simulink model "overalldesign_change_down"  (R2025b)
settings: Solver=ode4  StartTime=0.0  StopTime=1200  FixedStep=0.01  MaxStep=0.01  RelTol=1e-4
PreLoadFcn:
  | % Component data matrix: [present, weight_kg, MX_kgmm, MY_kgmm, MZ_kgmm]
  | % Rows 1-28 correspond to Excel rows 2-29
  | comp_data_mat = [
  |   1, 80,     147543.64,  -0.88,    -1622.36;    % 底盘
  |   1, 60,      73274.04, -169.26,    3359.46;    % 轮胎
  |   0,  0,             0,       0,         0;    % 前后桥(不在位)
  |   1, 45,      99639.05,  -0.495,   35241.39;    % 蒙皮
  |   1, 159,    308512.15, -0.0298,   72044.97;    % 结构骨架
  |   1, 93,     214584.20,  -1.023,   85225.94;    % 折叠机构
  |   1, 113.92, 269830.46, -1.2531,  107552.44;    % 支臂
  |   1, 45,       1371.65, -531.27,   17662.14;    % 内饰
  |   1, 13.86,   34638.76, -0.1525,   13254.18;    % 电机底座
  |   1, 30,      69816.09,   -0.33,   26989.32;    % 飞行体
  |   1, 316,    803427.47,       0,   33092.78;    % 动力电池1
  |   0, 316,            0,       0,         0;    % 动力电池2(不在位)
  |   1, 30,      75059.94,    0.21,   37410.81;    % 旋翼
  |   1, 141,    353019.16,  -1.551,  161459.10;    % 电机
  |   1, 33,      82253.26,   -0.33,   27077.13;    % 电调
  |   1, 15,             0,       0,         0;    % PDU
  |   0, 10,             0,       0,         0;    % 导线(不在位)
  |   0,  0,             0,       0,         0;    % (空)
  |   0, 90,             0,       0,         0;    % 左商载(不在位)
  |   0, 90,             0,       0,         0;    % 右商载(不在位)
  |   0, 32,             0,       0,         0;    % 飞控运控(不在位)
  | 
  | ];
  | % Lift center [X; Y; Z] in mm
  | lift_center_vec = [2506.477; 0; 1258.273];
  | % Route parameters are set directly in top-level Constant blocks:
  | %   route_mode, takeoff, hover, line_cruise, circle_cruise, land
model workspace (MAT data in the model file):
  CS_duct_lift_slew_rate = 7031250
  CS_main_rotor_slew_rate = 1567.1641791
  CS_max_acc_xy = 5
  CS_max_acc_z_down = 5
  CS_max_acc_z_up = 5
  CS_max_jerk_xy = 20
  CS_max_jerk_z_down = 20
  CS_max_jerk_z_up = 20
  CS_max_vel_xy = 20
  CS_max_vel_z_down = 20
  CS_max_vel_z_up = 20
  CS_motor_tau_duct = 0.07
  CS_motor_tau_main = 0.336
  Kd_rate_rp = 12
  Kd_rate_y = 8
  Kd_vel_xy = 1.5
  Kd_vel_z = 1
  Ki_rate_rp = 4
  Ki_rate_y = 10
  Ki_vel_xy = 0.02
  Ki_vel_z = 0.05
  Kp_att_rp = 2.5
  Kp_att_tilt = 2.5
  Kp_att_y = 1.5
  Kp_att_yaw = 1.5
  Kp_pos_xy = 0.4
  Kp_pos_z = 1
  Kp_rate_rp = 300
  Kp_rate_y = 200
  Kp_vel_xy = 1.5
  Kp_vel_z = 1.5
  P : object (value not decoded)
  T_hover = 11772
  V_descent = []
  W_hover = 1194
  W_margin = 1600
  cg_offset_m = [0.038293; -0.0063; 0.28227]
  cg_x_delta_m = 0
  climbRate_mps = 5
  cruiseSpeed_mps = 20
  descentRate_mps = 5
  duct_dir = [0  -1  0; 0  1  0]
  duct_pos_0 = [3  0  0; 3  0  0]
  fault_id = 0
  fault_mask = [0; 0; 0; 0; 0; 0; 0; 0]
  hover_x = 0
  hover_y = 0
  hover_yaw = 0
  hover_z = -120
  inertia_kgm2 = [3959.6  0  0; 0  3041.4  0; 0  0  2640.2]
  kF = 0.0013767
  kF_duct = 4.54e-05
  kM = 0.000164967
  kM_coeff = 1.72621225e-05
  kM_duct = 4.896e-06
  kM_duct_coeff = 5.12708e-07
  k_yaw_weight = 0.5
  mass_kg = 1200
  motor_coord = [2.624 2.624 0 0 -2.599 -2.599 3 3 -2.228 2.228 -2.235 2.235 ... (24 elements, 8x3)]
  motor_dir = [1; -1; -1; 1; 1; -1]
  motor_efficiency = 0.9016
  motor_pos_0 = [2.624 2.624 0 0 -2.599 -2.599 -2.228 2.228 -2.235 2.235 -2.231 2.231 ... (18 elements, 6x3)]
  offline_opt_applyBestToModel = 1
  offline_opt_maxEvaluations = 10
  offline_opt_method = 'auto'
  offline_opt_saveBestToModel = 0
  offline_opt_updateDiagramAfterBest = 1
  perf_battery_Wh = 80000
  perf_blade_num = 2
  perf_chord_avg = 0.18
  perf_mass_kg = 1200
  perf_rho = 1.225
  perf_rotor_num = 6
  perf_rotor_radius = 1.3
  perf_usable_ratio = 0.8
  speed_max_radps = 1750
  tau_limit_rp = 2000
  tau_limit_y = 1000
  thrust_degrade = 0.7
libraries: slpidlib x6, aerolibprivatev1p5 x1, dspnetwork x1
(part 2 of 2)

== system overalldesign_change_down/Flight_Simulation/controller/Rate_Controller ==
  p_sp : Inport
  q_sp : Inport  Port=2
  r_sp : Inport  Port=3
  cur_p : Inport  Port=4
  cur_q : Inport  Port=5
  cur_r : Inport  Port=6
  PID_RatePitch : slpidlib/PID Controller  Controller=PID  Form=Parallel  TimeDomain=Continuous-time  UseExternalTs=off  SampleTime=-1  IntegratorMethod=Forward Euler  FilterMethod=Forward Euler  ControllerParametersSource=internal  P=Kp_rate_rp  I=Ki_rate_rp  UseKiTs=off  D=Kd_rate_rp  UseExternalDerivativeSource=off  N=100  UseFilter=on  TunerSelectOption=Transfer Function Based (PID Tuner App)  InitialConditionSource=internal  InitialConditionForIntegrator=0  InitialConditionForFilter=0  DifferentiatorICPrevScaledInput=0  ExternalReset=none  TrackingMode=off  Kt=1  LimitOutput=on  SatLimitsSource=internal  UpperSaturationLimit=tau_limit_rp  LowerSaturationLimit=-tau_limit_rp  LinearizeAsGain=on  AntiWindupMode=clamping  Kb=1  LimitIntegrator=on  UpperIntegratorSaturationLimit=tau_limit_rp  LowerIntegratorSaturationLimit=-tau_limit_rp  POutMin=[]  POutMax=[]  IOutMin=[]  IOutMax=[]  DOutMin=[]  DOutMax=[]  NOutMin=[]  NOutMax=[]  SumOutMin=[]  SumOutMax=[]  SaturationOutMin=[]  SaturationOutMax=[]  PParamMin=[]  PParamMax=[]  IParamMin=[]  IParamMax=[]  DParamMin=[]  DParamMax=[]  NParamMin=[]  NParamMax=[]  KbParamMin=[]  KbParamMax=[]  KtParamMin=[]  KtParamMax=[]  KbOutMin=[]  KbOutMax=[]  KtOutMin=[]  KtOutMax=[]  IntegratorOutMin=[]  IntegratorOutMax=[]  FilterOutMin=[]  FilterOutMax=[]  SumI1OutMin=[]  SumI1OutMax=[]  SumI2OutMin=[]  SumI2OutMax=[]  SumI3OutMin=[]  SumI3OutMax=[]  SumI4OutMin=[]  SumI4OutMax=[]  SumDOutMin=[]  SumDOutMax=[]  DifferentiatorOutMin=[]  DifferentiatorOutMax=[]  FilterDiffOutCoefMin=[]  FilterDiffOutCoefMax=[]  ReciprocalOutMin=[]  ReciprocalOutMax=[]  SumDenOutMin=[]  SumDenOutMax=[]  SumNumOutMin=[]  SumNumOutMax=[]  DivideOutMin=[]  DivideOutMax=[]  UdiffTsProdOutMin=[]  UdiffTsProdOutMax=[]  NTsProdOutMin=[]  NTsProdOutMax=[]  UintegralTsProdOutMin=[]  UintegralTsProdOutMax=[]  UngainTsProdOutMin=[]  UngainTsProdOutMax=[]  ClampingZeroOutDataTypeStr=Inherit: Inherit via back propagation  ClampingZeroOutMin=[]  ClampingZeroOutMax=[]  FilterDenConstantOutDataTypeStr=Inherit: Inherit via back propagation  FilterDenConstantOutMin=[]  FilterDenConstantOutMax=[]  PCopyOutDataTypeStr=Inherit: Inherit via back propagation  PCopyOutMin=[]  PCopyOutMax=[]  NCopyOutDataTypeStr=Inherit: Inherit via back propagation  NCopyOutMin=[]  NCopyOutMax=[]  IntegratorContinuousStateAttributes=''  IntegratorStateMustResolveToSignalObject=off  IntegratorRTWStateStorageClass=Auto  FilterContinuousStateAttributes=''  FilterStateMustResolveToSignalObject=off  FilterRTWStateStorageClass=Auto  ParallelPVariant=InternalParameters  IdealPVariant=Disabled  IVariant=InternalParameters  DVariant=InternalParameters  IntegratorVariant=Continuous  SatVariant=Enabled  AWVariant=ContClampingParallel  PCopyVariant=Disabled  TRVariant=Disabled  FdbkBlocksVariant=Forward  IdealPFdbkVariant=Disabled  SatFdbkVariant=Disabled  DerivativeFilterVariant=ContFilter  NVariant=InternalParameters  NCopyVariant=Disabled  FilterICVariant=InternalICsFilter  IntegratorICVariant=InternalICs  ExternalResetVariant=Disabled  TRSumVariant=Passthrough  SumFdbkVariant=Disabled  SumVariant=Sum_PID  TsampFilterVariant=InternalTs  TsampNgainVariant=Passthrough  TsampIntegralVariant=Disabled_SignalSpec  ExternalSaturationOutDataTypeStr=Inherit: Same as second input  DerivativeSourceVariant=ErrorSignal  PreIntVariant=InternalPreInt
  PID_RateRoll : slpidlib/PID Controller  Controller=PID  Form=Parallel  TimeDomain=Continuous-time  UseExternalTs=off  SampleTime=-1  IntegratorMethod=Forward Euler  FilterMethod=Forward Euler  ControllerParametersSource=internal  P=Kp_rate_rp  I=Ki_rate_rp  UseKiTs=off  D=Kd_rate_rp  UseExternalDerivativeSource=off  N=100  UseFilter=on  TunerSelectOption=Transfer Function Based (PID Tuner App)  InitialConditionSource=internal  InitialConditionForIntegrator=0  InitialConditionForFilter=0  DifferentiatorICPrevScaledInput=0  ExternalReset=none  TrackingMode=off  Kt=1  LimitOutput=on  SatLimitsSource=internal  UpperSaturationLimit=tau_limit_rp  LowerSaturationLimit=-tau_limit_rp  LinearizeAsGain=on  AntiWindupMode=clamping  Kb=1  LimitIntegrator=on  UpperIntegratorSaturationLimit=tau_limit_rp  LowerIntegratorSaturationLimit=-tau_limit_rp  POutMin=[]  POutMax=[]  IOutMin=[]  IOutMax=[]  DOutMin=[]  DOutMax=[]  NOutMin=[]  NOutMax=[]  SumOutMin=[]  SumOutMax=[]  SaturationOutMin=[]  SaturationOutMax=[]  PParamMin=[]  PParamMax=[]  IParamMin=[]  IParamMax=[]  DParamMin=[]  DParamMax=[]  NParamMin=[]  NParamMax=[]  KbParamMin=[]  KbParamMax=[]  KtParamMin=[]  KtParamMax=[]  KbOutMin=[]  KbOutMax=[]  KtOutMin=[]  KtOutMax=[]  IntegratorOutMin=[]  IntegratorOutMax=[]  FilterOutMin=[]  FilterOutMax=[]  SumI1OutMin=[]  SumI1OutMax=[]  SumI2OutMin=[]  SumI2OutMax=[]  SumI3OutMin=[]  SumI3OutMax=[]  SumI4OutMin=[]  SumI4OutMax=[]  SumDOutMin=[]  SumDOutMax=[]  DifferentiatorOutMin=[]  DifferentiatorOutMax=[]  FilterDiffOutCoefMin=[]  FilterDiffOutCoefMax=[]  ReciprocalOutMin=[]  ReciprocalOutMax=[]  SumDenOutMin=[]  SumDenOutMax=[]  SumNumOutMin=[]  SumNumOutMax=[]  DivideOutMin=[]  DivideOutMax=[]  UdiffTsProdOutMin=[]  UdiffTsProdOutMax=[]  NTsProdOutMin=[]  NTsProdOutMax=[]  UintegralTsProdOutMin=[]  UintegralTsProdOutMax=[]  UngainTsProdOutMin=[]  UngainTsProdOutMax=[]  ClampingZeroOutDataTypeStr=Inherit: Inherit via back propagation  ClampingZeroOutMin=[]  ClampingZeroOutMax=[]  FilterDenConstantOutDataTypeStr=Inherit: Inherit via back propagation  FilterDenConstantOutMin=[]  FilterDenConstantOutMax=[]  PCopyOutDataTypeStr=Inherit: Inherit via back propagation  PCopyOutMin=[]  PCopyOutMax=[]  NCopyOutDataTypeStr=Inherit: Inherit via back propagation  NCopyOutMin=[]  NCopyOutMax=[]  IntegratorContinuousStateAttributes=''  IntegratorStateMustResolveToSignalObject=off  IntegratorRTWStateStorageClass=Auto  FilterContinuousStateAttributes=''  FilterStateMustResolveToSignalObject=off  FilterRTWStateStorageClass=Auto  ParallelPVariant=InternalParameters  IdealPVariant=Disabled  IVariant=InternalParameters  DVariant=InternalParameters  IntegratorVariant=Continuous  SatVariant=Enabled  AWVariant=ContClampingParallel  PCopyVariant=Disabled  TRVariant=Disabled  FdbkBlocksVariant=Forward  IdealPFdbkVariant=Disabled  SatFdbkVariant=Disabled  DerivativeFilterVariant=ContFilter  NVariant=InternalParameters  NCopyVariant=Disabled  FilterICVariant=InternalICsFilter  IntegratorICVariant=InternalICs  ExternalResetVariant=Disabled  TRSumVariant=Passthrough  SumFdbkVariant=Disabled  SumVariant=Sum_PID  TsampFilterVariant=InternalTs  TsampNgainVariant=Passthrough  TsampIntegralVariant=Disabled_SignalSpec  ExternalSaturationOutDataTypeStr=Inherit: Same as second input  DerivativeSourceVariant=ErrorSignal  PreIntVariant=InternalPreInt
  PID_RateYaw : slpidlib/PID Controller  Controller=PID  Form=Parallel  TimeDomain=Continuous-time  UseExternalTs=off  SampleTime=-1  IntegratorMethod=Forward Euler  FilterMethod=Forward Euler  ControllerParametersSource=internal  P=Kp_rate_y  I=Ki_rate_y  UseKiTs=off  D=Kd_rate_y  UseExternalDerivativeSource=off  N=100  UseFilter=on  TunerSelectOption=Transfer Function Based (PID Tuner App)  InitialConditionSource=internal  InitialConditionForIntegrator=0  InitialConditionForFilter=0  DifferentiatorICPrevScaledInput=0  ExternalReset=none  TrackingMode=off  Kt=1  LimitOutput=on  SatLimitsSource=internal  UpperSaturationLimit=tau_limit_y  LowerSaturationLimit=-tau_limit_y  LinearizeAsGain=on  AntiWindupMode=clamping  Kb=1  LimitIntegrator=on  UpperIntegratorSaturationLimit=tau_limit_y  LowerIntegratorSaturationLimit=-tau_limit_y  POutMin=[]  POutMax=[]  IOutMin=[]  IOutMax=[]  DOutMin=[]  DOutMax=[]  NOutMin=[]  NOutMax=[]  SumOutMin=[]  SumOutMax=[]  SaturationOutMin=[]  SaturationOutMax=[]  PParamMin=[]  PParamMax=[]  IParamMin=[]  IParamMax=[]  DParamMin=[]  DParamMax=[]  NParamMin=[]  NParamMax=[]  KbParamMin=[]  KbParamMax=[]  KtParamMin=[]  KtParamMax=[]  KbOutMin=[]  KbOutMax=[]  KtOutMin=[]  KtOutMax=[]  IntegratorOutMin=[]  IntegratorOutMax=[]  FilterOutMin=[]  FilterOutMax=[]  SumI1OutMin=[]  SumI1OutMax=[]  SumI2OutMin=[]  SumI2OutMax=[]  SumI3OutMin=[]  SumI3OutMax=[]  SumI4OutMin=[]  SumI4OutMax=[]  SumDOutMin=[]  SumDOutMax=[]  DifferentiatorOutMin=[]  DifferentiatorOutMax=[]  FilterDiffOutCoefMin=[]  FilterDiffOutCoefMax=[]  ReciprocalOutMin=[]  ReciprocalOutMax=[]  SumDenOutMin=[]  SumDenOutMax=[]  SumNumOutMin=[]  SumNumOutMax=[]  DivideOutMin=[]  DivideOutMax=[]  UdiffTsProdOutMin=[]  UdiffTsProdOutMax=[]  NTsProdOutMin=[]  NTsProdOutMax=[]  UintegralTsProdOutMin=[]  UintegralTsProdOutMax=[]  UngainTsProdOutMin=[]  UngainTsProdOutMax=[]  ClampingZeroOutDataTypeStr=Inherit: Inherit via back propagation  ClampingZeroOutMin=[]  ClampingZeroOutMax=[]  FilterDenConstantOutDataTypeStr=Inherit: Inherit via back propagation  FilterDenConstantOutMin=[]  FilterDenConstantOutMax=[]  PCopyOutDataTypeStr=Inherit: Inherit via back propagation  PCopyOutMin=[]  PCopyOutMax=[]  NCopyOutDataTypeStr=Inherit: Inherit via back propagation  NCopyOutMin=[]  NCopyOutMax=[]  IntegratorContinuousStateAttributes=''  IntegratorStateMustResolveToSignalObject=off  IntegratorRTWStateStorageClass=Auto  FilterContinuousStateAttributes=''  FilterStateMustResolveToSignalObject=off  FilterRTWStateStorageClass=Auto  ParallelPVariant=InternalParameters  IdealPVariant=Disabled  IVariant=InternalParameters  DVariant=InternalParameters  IntegratorVariant=Continuous  SatVariant=Enabled  AWVariant=ContClampingParallel  PCopyVariant=Disabled  TRVariant=Disabled  FdbkBlocksVariant=Forward  IdealPFdbkVariant=Disabled  SatFdbkVariant=Disabled  DerivativeFilterVariant=ContFilter  NVariant=InternalParameters  NCopyVariant=Disabled  FilterICVariant=InternalICsFilter  IntegratorICVariant=InternalICs  ExternalResetVariant=Disabled  TRSumVariant=Passthrough  SumFdbkVariant=Disabled  SumVariant=Sum_PID  TsampFilterVariant=InternalTs  TsampNgainVariant=Passthrough  TsampIntegralVariant=Disabled_SignalSpec  ExternalSaturationOutDataTypeStr=Inherit: Same as second input  DerivativeSourceVariant=ErrorSignal  PreIntVariant=InternalPreInt
  Sum_Pitch : Sum  Inputs=+-
  Sum_Roll : Sum  Inputs=+-
  Sum_Yaw : Sum  Inputs=+-
  tau_x : Outport
  tau_y : Outport  Port=2
  tau_z : Outport  Port=3
  wires:
  Sum_Yaw/1 -> PID_RateYaw/1
  p_sp/1 -> Sum_Roll/1
  cur_q/1 -> Sum_Pitch/2
  cur_p/1 -> Sum_Roll/2
  PID_RateYaw/1 -> tau_z/1
  r_sp/1 -> Sum_Yaw/1
  cur_r/1 -> Sum_Yaw/2
  q_sp/1 -> Sum_Pitch/1
  Sum_Roll/1 -> PID_RateRoll/1
  Sum_Pitch/1 -> PID_RatePitch/1
  PID_RateRoll/1 -> tau_x/1
  PID_RatePitch/1 -> tau_y/1

== system overalldesign_change_down/Flight_Simulation/controller/Velocity_Controller ==
  vx_sp : Inport
  vy_sp : Inport  Port=2
  vz_sp : Inport  Port=3
  cur_vx : Inport  Port=4
  cur_vy : Inport  Port=5
  cur_vz : Inport  Port=6
  AccelJerkLimit_X : RateLimiter  RisingSlewLimit=CS_max_jerk_xy  FallingSlewLimit=-CS_max_jerk_xy  SampleTimeMode=inherited
  AccelJerkLimit_Y : RateLimiter  RisingSlewLimit=CS_max_jerk_xy  FallingSlewLimit=-CS_max_jerk_xy  SampleTimeMode=inherited
  AccelJerkLimit_Z : RateLimiter  RisingSlewLimit=CS_max_jerk_z_up  FallingSlewLimit=-CS_max_jerk_z_down  SampleTimeMode=inherited
  PID_VelX : slpidlib/PID Controller  Controller=PID  Form=Parallel  TimeDomain=Continuous-time  UseExternalTs=off  SampleTime=-1  IntegratorMethod=Forward Euler  FilterMethod=Forward Euler  ControllerParametersSource=internal  P=Kp_vel_xy  I=Ki_vel_xy  UseKiTs=off  D=Kd_vel_xy  UseExternalDerivativeSource=off  N=10  UseFilter=on  TunerSelectOption=Transfer Function Based (PID Tuner App)  InitialConditionSource=internal  InitialConditionForIntegrator=0  InitialConditionForFilter=0  DifferentiatorICPrevScaledInput=0  ExternalReset=none  TrackingMode=off  Kt=1  LimitOutput=on  SatLimitsSource=internal  UpperSaturationLimit=CS_max_acc_xy  LowerSaturationLimit=-CS_max_acc_xy  LinearizeAsGain=on  AntiWindupMode=clamping  Kb=1  LimitIntegrator=on  UpperIntegratorSaturationLimit=5  LowerIntegratorSaturationLimit=-5  POutMin=[]  POutMax=[]  IOutMin=[]  IOutMax=[]  DOutMin=[]  DOutMax=[]  NOutMin=[]  NOutMax=[]  SumOutMin=[]  SumOutMax=[]  SaturationOutMin=[]  SaturationOutMax=[]  PParamMin=[]  PParamMax=[]  IParamMin=[]  IParamMax=[]  DParamMin=[]  DParamMax=[]  NParamMin=[]  NParamMax=[]  KbParamMin=[]  KbParamMax=[]  KtParamMin=[]  KtParamMax=[]  KbOutMin=[]  KbOutMax=[]  KtOutMin=[]  KtOutMax=[]  IntegratorOutMin=[]  IntegratorOutMax=[]  FilterOutMin=[]  FilterOutMax=[]  SumI1OutMin=[]  SumI1OutMax=[]  SumI2OutMin=[]  SumI2OutMax=[]  SumI3OutMin=[]  SumI3OutMax=[]  SumI4OutMin=[]  SumI4OutMax=[]  SumDOutMin=[]  SumDOutMax=[]  DifferentiatorOutMin=[]  DifferentiatorOutMax=[]  FilterDiffOutCoefMin=[]  FilterDiffOutCoefMax=[]  ReciprocalOutMin=[]  ReciprocalOutMax=[]  SumDenOutMin=[]  SumDenOutMax=[]  SumNumOutMin=[]  SumNumOutMax=[]  DivideOutMin=[]  DivideOutMax=[]  UdiffTsProdOutMin=[]  UdiffTsProdOutMax=[]  NTsProdOutMin=[]  NTsProdOutMax=[]  UintegralTsProdOutMin=[]  UintegralTsProdOutMax=[]  UngainTsProdOutMin=[]  UngainTsProdOutMax=[]  ClampingZeroOutDataTypeStr=Inherit: Inherit via back propagation  ClampingZeroOutMin=[]  ClampingZeroOutMax=[]  FilterDenConstantOutDataTypeStr=Inherit: Inherit via back propagation  FilterDenConstantOutMin=[]  FilterDenConstantOutMax=[]  PCopyOutDataTypeStr=Inherit: Inherit via back propagation  PCopyOutMin=[]  PCopyOutMax=[]  NCopyOutDataTypeStr=Inherit: Inherit via back propagation  NCopyOutMin=[]  NCopyOutMax=[]  IntegratorContinuousStateAttributes=''  IntegratorStateMustResolveToSignalObject=off  IntegratorRTWStateStorageClass=Auto  FilterContinuousStateAttributes=''  FilterStateMustResolveToSignalObject=off  FilterRTWStateStorageClass=Auto  ParallelPVariant=InternalParameters  IdealPVariant=Disabled  IVariant=InternalParameters  DVariant=InternalParameters  IntegratorVariant=Continuous  SatVariant=Enabled  AWVariant=ContClampingParallel  PCopyVariant=Disabled  TRVariant=Disabled  FdbkBlocksVariant=Forward  IdealPFdbkVariant=Disabled  SatFdbkVariant=Disabled  DerivativeFilterVariant=ContFilter  NVariant=InternalParameters  NCopyVariant=Disabled  FilterICVariant=InternalICsFilter  IntegratorICVariant=InternalICs  ExternalResetVariant=Disabled  TRSumVariant=Passthrough  SumFdbkVariant=Disabled  SumVariant=Sum_PID  TsampFilterVariant=InternalTs  TsampNgainVariant=Passthrough  TsampIntegralVariant=Disabled_SignalSpec  ExternalSaturationOutDataTypeStr=Inherit: Same as second input  DerivativeSourceVariant=ErrorSignal  PreIntVariant=InternalPreInt
  PID_VelY : slpidlib/PID Controller  Controller=PID  Form=Parallel  TimeDomain=Continuous-time  UseExternalTs=off  SampleTime=-1  IntegratorMethod=Forward Euler  FilterMethod=Forward Euler  ControllerParametersSource=internal  P=Kp_vel_xy  I=Ki_vel_xy  UseKiTs=off  D=Kd_vel_xy  UseExternalDerivativeSource=off  N=10  UseFilter=on  TunerSelectOption=Transfer Function Based (PID Tuner App)  InitialConditionSource=internal  InitialConditionForIntegrator=0  InitialConditionForFilter=0  DifferentiatorICPrevScaledInput=0  ExternalReset=none  TrackingMode=off  Kt=1  LimitOutput=on  SatLimitsSource=internal  UpperSaturationLimit=CS_max_acc_xy  LowerSaturationLimit=-CS_max_acc_xy  LinearizeAsGain=on  AntiWindupMode=clamping  Kb=1  LimitIntegrator=on  UpperIntegratorSaturationLimit=5  LowerIntegratorSaturationLimit=-5  POutMin=[]  POutMax=[]  IOutMin=[]  IOutMax=[]  DOutMin=[]  DOutMax=[]  NOutMin=[]  NOutMax=[]  SumOutMin=[]  SumOutMax=[]  SaturationOutMin=[]  SaturationOutMax=[]  PParamMin=[]  PParamMax=[]  IParamMin=[]  IParamMax=[]  DParamMin=[]  DParamMax=[]  NParamMin=[]  NParamMax=[]  KbParamMin=[]  KbParamMax=[]  KtParamMin=[]  KtParamMax=[]  KbOutMin=[]  KbOutMax=[]  KtOutMin=[]  KtOutMax=[]  IntegratorOutMin=[]  IntegratorOutMax=[]  FilterOutMin=[]  FilterOutMax=[]  SumI1OutMin=[]  SumI1OutMax=[]  SumI2OutMin=[]  SumI2OutMax=[]  SumI3OutMin=[]  SumI3OutMax=[]  SumI4OutMin=[]  SumI4OutMax=[]  SumDOutMin=[]  SumDOutMax=[]  DifferentiatorOutMin=[]  DifferentiatorOutMax=[]  FilterDiffOutCoefMin=[]  FilterDiffOutCoefMax=[]  ReciprocalOutMin=[]  ReciprocalOutMax=[]  SumDenOutMin=[]  SumDenOutMax=[]  SumNumOutMin=[]  SumNumOutMax=[]  DivideOutMin=[]  DivideOutMax=[]  UdiffTsProdOutMin=[]  UdiffTsProdOutMax=[]  NTsProdOutMin=[]  NTsProdOutMax=[]  UintegralTsProdOutMin=[]  UintegralTsProdOutMax=[]  UngainTsProdOutMin=[]  UngainTsProdOutMax=[]  ClampingZeroOutDataTypeStr=Inherit: Inherit via back propagation  ClampingZeroOutMin=[]  ClampingZeroOutMax=[]  FilterDenConstantOutDataTypeStr=Inherit: Inherit via back propagation  FilterDenConstantOutMin=[]  FilterDenConstantOutMax=[]  PCopyOutDataTypeStr=Inherit: Inherit via back propagation  PCopyOutMin=[]  PCopyOutMax=[]  NCopyOutDataTypeStr=Inherit: Inherit via back propagation  NCopyOutMin=[]  NCopyOutMax=[]  IntegratorContinuousStateAttributes=''  IntegratorStateMustResolveToSignalObject=off  IntegratorRTWStateStorageClass=Auto  FilterContinuousStateAttributes=''  FilterStateMustResolveToSignalObject=off  FilterRTWStateStorageClass=Auto  ParallelPVariant=InternalParameters  IdealPVariant=Disabled  IVariant=InternalParameters  DVariant=InternalParameters  IntegratorVariant=Continuous  SatVariant=Enabled  AWVariant=ContClampingParallel  PCopyVariant=Disabled  TRVariant=Disabled  FdbkBlocksVariant=Forward  IdealPFdbkVariant=Disabled  SatFdbkVariant=Disabled  DerivativeFilterVariant=ContFilter  NVariant=InternalParameters  NCopyVariant=Disabled  FilterICVariant=InternalICsFilter  IntegratorICVariant=InternalICs  ExternalResetVariant=Disabled  TRSumVariant=Passthrough  SumFdbkVariant=Disabled  SumVariant=Sum_PID  TsampFilterVariant=InternalTs  TsampNgainVariant=Passthrough  TsampIntegralVariant=Disabled_SignalSpec  ExternalSaturationOutDataTypeStr=Inherit: Same as second input  DerivativeSourceVariant=ErrorSignal  PreIntVariant=InternalPreInt
  PID_VelZ : slpidlib/PID Controller  Controller=PID  Form=Parallel  TimeDomain=Continuous-time  UseExternalTs=off  SampleTime=-1  IntegratorMethod=Forward Euler  FilterMethod=Forward Euler  ControllerParametersSource=internal  P=Kp_vel_z  I=Ki_vel_z  UseKiTs=off  D=Kd_vel_z  UseExternalDerivativeSource=off  N=10  UseFilter=on  TunerSelectOption=Transfer Function Based (PID Tuner App)  InitialConditionSource=internal  InitialConditionForIntegrator=0  InitialConditionForFilter=0  DifferentiatorICPrevScaledInput=0  ExternalReset=none  TrackingMode=off  Kt=1  LimitOutput=on  SatLimitsSource=internal  UpperSaturationLimit=CS_max_acc_z_up  LowerSaturationLimit=-CS_max_acc_z_down  LinearizeAsGain=on  AntiWindupMode=clamping  Kb=1  LimitIntegrator=on  UpperIntegratorSaturationLimit=5  LowerIntegratorSaturationLimit=-5  POutMin=[]  POutMax=[]  IOutMin=[]  IOutMax=[]  DOutMin=[]  DOutMax=[]  NOutMin=[]  NOutMax=[]  SumOutMin=[]  SumOutMax=[]  SaturationOutMin=[]  SaturationOutMax=[]  PParamMin=[]  PParamMax=[]  IParamMin=[]  IParamMax=[]  DParamMin=[]  DParamMax=[]  NParamMin=[]  NParamMax=[]  KbParamMin=[]  KbParamMax=[]  KtParamMin=[]  KtParamMax=[]  KbOutMin=[]  KbOutMax=[]  KtOutMin=[]  KtOutMax=[]  IntegratorOutMin=[]  IntegratorOutMax=[]  FilterOutMin=[]  FilterOutMax=[]  SumI1OutMin=[]  SumI1OutMax=[]  SumI2OutMin=[]  SumI2OutMax=[]  SumI3OutMin=[]  SumI3OutMax=[]  SumI4OutMin=[]  SumI4OutMax=[]  SumDOutMin=[]  SumDOutMax=[]  DifferentiatorOutMin=[]  DifferentiatorOutMax=[]  FilterDiffOutCoefMin=[]  FilterDiffOutCoefMax=[]  ReciprocalOutMin=[]  ReciprocalOutMax=[]  SumDenOutMin=[]  SumDenOutMax=[]  SumNumOutMin=[]  SumNumOutMax=[]  DivideOutMin=[]  DivideOutMax=[]  UdiffTsProdOutMin=[]  UdiffTsProdOutMax=[]  NTsProdOutMin=[]  NTsProdOutMax=[]  UintegralTsProdOutMin=[]  UintegralTsProdOutMax=[]  UngainTsProdOutMin=[]  UngainTsProdOutMax=[]  ClampingZeroOutDataTypeStr=Inherit: Inherit via back propagation  ClampingZeroOutMin=[]  ClampingZeroOutMax=[]  FilterDenConstantOutDataTypeStr=Inherit: Inherit via back propagation  FilterDenConstantOutMin=[]  FilterDenConstantOutMax=[]  PCopyOutDataTypeStr=Inherit: Inherit via back propagation  PCopyOutMin=[]  PCopyOutMax=[]  NCopyOutDataTypeStr=Inherit: Inherit via back propagation  NCopyOutMin=[]  NCopyOutMax=[]  IntegratorContinuousStateAttributes=''  IntegratorStateMustResolveToSignalObject=off  IntegratorRTWStateStorageClass=Auto  FilterContinuousStateAttributes=''  FilterStateMustResolveToSignalObject=off  FilterRTWStateStorageClass=Auto  ParallelPVariant=InternalParameters  IdealPVariant=Disabled  IVariant=InternalParameters  DVariant=InternalParameters  IntegratorVariant=Continuous  SatVariant=Enabled  AWVariant=ContClampingParallel  PCopyVariant=Disabled  TRVariant=Disabled  FdbkBlocksVariant=Forward  IdealPFdbkVariant=Disabled  SatFdbkVariant=Disabled  DerivativeFilterVariant=ContFilter  NVariant=InternalParameters  NCopyVariant=Disabled  FilterICVariant=InternalICsFilter  IntegratorICVariant=InternalICs  ExternalResetVariant=Disabled  TRSumVariant=Passthrough  SumFdbkVariant=Disabled  SumVariant=Sum_PID  TsampFilterVariant=InternalTs  TsampNgainVariant=Passthrough  TsampIntegralVariant=Disabled_SignalSpec  ExternalSaturationOutDataTypeStr=Inherit: Same as second input  DerivativeSourceVariant=ErrorSignal  PreIntVariant=InternalPreInt
  Sum_X : Sum  Inputs=+-
  Sum_Y : Sum  Inputs=+-
  Sum_Z : Sum  Inputs=+-
  ax_sp : Outport
  ay_sp : Outport  Port=2
  az_sp : Outport  Port=3
  wires:
  Sum_X/1 -> PID_VelX/1
  vx_sp/1 -> Sum_X/1
  cur_vy/1 -> Sum_Y/2
  cur_vz/1 -> Sum_Z/2
  vz_sp/1 -> Sum_Z/1
  cur_vx/1 -> Sum_X/2
  Sum_Z/1 -> PID_VelZ/1
  vy_sp/1 -> Sum_Y/1
  Sum_Y/1 -> PID_VelY/1
  PID_VelX/1 -> AccelJerkLimit_X/1
  AccelJerkLimit_X/1 -> ax_sp/1
  PID_VelY/1 -> AccelJerkLimit_Y/1
  AccelJerkLimit_Y/1 -> ay_sp/1
  PID_VelZ/1 -> AccelJerkLimit_Z/1
  AccelJerkLimit_Z/1 -> az_sp/1

== matlab function overalldesign_change_down/Flight_Simulation/mixer/mixer_fcn ==
  data: T_des input; W output; tau_y input; tau_x input; tau_z input; fault_id input; CGoffset input size=3; motor_coord input
function W = fcn(T_des, tau_y, tau_x, tau_z, fault_id, CGoffset, motor_coord)
kF = 0.0013767; kM = 0.000164967; kF_duct = 4.54e-05;
T_hover = 11772; W_hover = sqrt((T_hover / 6) / kF);

motor_X = motor_coord(1:6, 1);
motor_Y = motor_coord(1:6, 2);
duct_X = motor_coord(7:8, 1);
motor_dir = [1; -1; -1; 1; 1; -1];

M0_col_norms = [2.0417; 2.1786; 2.5193; 2.4934];

CGx = CGoffset(1); CGy = CGoffset(2);
arm_pitch = motor_X - CGx;
arm_roll  = motor_Y - CGy;
duct_arm_x = duct_X - CGx;

healthy = ones(8,1);
if fault_id > 0 && fault_id <= 8
    healthy(fault_id) = 0;
end

% Trim: analytic for healthy, QP for fault
if fault_id == 0
    T_target = max(T_des, 1000) / kF;
    Feq = T_target / 6;
    pitch_per_rotor = arm_pitch(1) + arm_pitch(3) + arm_pitch(5);
    pitch_err = Feq * pitch_per_rotor * 2;
    k1 = -pitch_err / (2*(arm_pitch(1) - arm_pitch(5)));
    Ff = Feq + k1; Fm = Feq; Fr = Feq - k1;
    W_trim = zeros(8,1);
    W_trim(1:2) = sqrt(max(1, Ff));
    W_trim(3:4) = sqrt(max(1, Fm));
    W_trim(5:6) = sqrt(max(1, Fr));
    W_trim(7:8) = 0;
    W_trim = min(1750, max(0, W_trim));
else
    n_act_rotors = sum(healthy(1:6));
    W_margin = 1600;
    T_cap = n_act_rotors * kF * W_margin^2 + 2 * kF_duct * W_margin^2;
    T_des_capped = min(T_des, T_cap * 0.86);
    full_idx = find(healthy); m_actuators = length(full_idx);
    A_full = zeros(4, m_actuators);
    for j = 1:m_actuators
        i = full_idx(j);
        if i <= 6
            A_full(1,j) = 1; A_full(2,j) = -arm_roll(i);
            A_full(3,j) = arm_pitch(i); A_full(4,j) = motor_dir(i) * kM / kF;
        else
            if i == 7
                A_full(4,j) = duct_arm_x(1) * kF_duct / kF;
            else
                A_full(4,j) = -duct_arm_x(2) * kF_duct / kF;
            end
        end
    end
    b = [T_des_capped / kF; 0; 0; 0];
    x = zeros(m_actuators, 1);
    active = true(m_actuators, 1); con_active = true(4, 1);
    reg_con = [1e-6, 5, 5, 1e-6];
    for iter = 1:8
        act_idx = find(active); m_act = length(act_idx);
        con_idx = find(con_active); n_con = length(con_idx);
        if m_act == 0 || n_con == 0
            break;
        end
        if n_con > m_act
            for c = 4:-1:1
                if con_active(c)
                    con_active(c) = false;
                    break;
                end
            end
            continue;
        end
        b_adj = b(con_idx);
        fi = find(~active);
        for jj = 1:length(fi)
            b_adj = b_adj - A_full(con_idx, fi(jj)) * x(fi(jj));
        end
        A_act = A_full(con_idx, act_idx);
        x0_a = W_hover^2 * ones(m_act, 1);
        x_act = x0_a - A_act' * pinv(A_act * A_act' + diag(reg_con(con_idx))) * (A_act * x0_a - b_adj);
        any_clamped = false;
        for jj = 1:m_act
            if x_act(jj) < 1
                x(act_idx(jj)) = 1;
                active(act_idx(jj)) = false;
                any_clamped = true;
            elseif x_act(jj) > 1750^2
                x(act_idx(jj)) = 1750^2;
                active(act_idx(jj)) = false;
                any_clamped = true;
            end
        end
        if ~any_clamped
            x(act_idx) = x_act;
            break;
        end
        if sum(active) < sum(con_active)
            for c = 4:-1:1
                if con_active(c)
                    con_active(c) = false;
                    break;
                end
            end
        end
    end
    W_trim = zeros(8,1);
    for j = 1:m_actuators
        W_trim(full_idx(j)) = sqrt(max(1, min(1750^2, x(j))));
    end
end

if fault_id > 0 && fault_id <= 8
    W_trim(fault_id) = 0;
end

% Compute M_phys at trim
G = zeros(4, 8);
for i = 1:8
    if W_trim(i) > 10
        if i <= 6
            dFdW = 2 * kF * W_trim(i);
            G(1,i) = dFdW; G(2,i) = arm_pitch(i) * dFdW;
            G(3,i) = -arm_roll(i) * dFdW; G(4,i) = motor_dir(i) * 2 * kM * W_trim(i);
        else
            dFdW = 2 * kF_duct * W_trim(i);
            if i == 7
                G(4,i) = duct_arm_x(1) * dFdW;
            else
                G(4,i) = -duct_arm_x(2) * dFdW;
            end
        end
    end
end
GGt = G * G';
M_phys = G' / (GGt + 1e-4*norm(GGt) * eye(4));
for c = 1:4
    hr_scale = 1.0;
    for i = 1:8
        if M_phys(i,c) > 1e-6 && W_trim(i) < 1750
            s = (1750 - W_trim(i)) / M_phys(i,c);
            hr_scale = min(hr_scale, max(0.1, s));
        elseif M_phys(i,c) < -1e-6 && W_trim(i) > 0
            s = W_trim(i) / (-M_phys(i,c));
            hr_scale = min(hr_scale, max(0.1, s));
        end
    end
    cn = norm(M_phys(:,c));
    if cn > 1e-10
        M_phys(:,c) = M_phys(:,c) * (M0_col_norms(c) / cn) * hr_scale;
    end
end

W = W_trim + M_phys * [0; tau_y; tau_x; tau_z];
if fault_id > 0 && fault_id <= 8
    W(fault_id) = 0;
end
W = min(1750, max(0, W));
end

== matlab function overalldesign_change_down/Route_Manager/Takeoff/smooth_takeoff ==
  data: t_clock input; z output; z_start input; z_target input; climb_rate input
function z = smooth_takeoff(t_clock, z_start, z_target, climb_rate)
t_accel = 8.0;
dz = z_target - z_start;
abs_dz = abs(dz);
if abs_dz < 0.01
    z = z_start;
else
    if t_clock <= t_accel
        progress = climb_rate * t_clock^2 / (2 * t_accel * abs_dz);
    else
        progress = climb_rate * (t_clock - t_accel/2) / abs_dz;
    end
    progress = max(0, min(1, progress));
    z = z_start + dz * progress;
end
end

== matlab function overalldesign_change_down/Route_Manager/Line_Cruise/smooth_cruise ==
  data: x output; t_clock input; y output; x0 input; y0 input; speed input; yaw input
function [x, y] = smooth_cruise(t_clock, x0, y0, speed, yaw)
t_clock = max(0, t_clock - 64);
t_accel = 8.0;
if t_clock <= t_accel
    s = 0.5 * speed / t_accel * t_clock^2;
else
    s = speed * (t_clock - t_accel/2);
end
x = x0 + s * cos(yaw);
y = y0 + s * sin(yaw);
end

== matlab function overalldesign_change_down/Flight_Simulation/Performance_Monitor/Perf_Calc ==
  data: t input; perf_vec output size=[20 1]; W input size=[8 1]; vel_world input size=[3 1]; P_mech input size=[8 1]; P_elec_total input size=1; Energy_Wh input size=1; perf_rho parameter double size=1; perf_mass_kg parameter double size=1; perf_rotor_num parameter double size=1; perf_rotor_radius parameter double size=1; perf_blade_num parameter double size=1; perf_chord_avg parameter double size=1; perf_battery_Wh parameter double size=1; perf_usable_ratio parameter double size=1
function perf_vec = Perf_Calc(t, W, vel_world, P_mech, P_elec_total, Energy_Wh, perf_rho, perf_mass_kg, perf_rotor_num, perf_rotor_radius, perf_blade_num, perf_chord_avg, perf_battery_Wh, perf_usable_ratio)
%#codegen
g = 9.81;
rho = perf_rho;
mass_kg = perf_mass_kg;
rotor_num = perf_rotor_num;
rotor_radius = perf_rotor_radius;% 这里换成真实旋翼半径
blade_num = perf_blade_num;% 这里换成单个旋翼桨叶数
chord_avg = perf_chord_avg; % 这里换成平均弦长
battery_Wh = perf_battery_Wh; % 这里换成真实电池容量
usable_ratio = perf_usable_ratio;
T = mass_kg * g;
A_total = rotor_num * pi * rotor_radius^2;
DL = T / max(A_total, 1e-6);
Vi = sqrt(DL / max(2 * rho, 1e-6));
Sigma = blade_num * chord_avg / max(pi * rotor_radius, 1e-6);
Pideal = T^(3/2) / max(sqrt(2 * rho * A_total), 1e-6);
P_mech_main = sum(P_mech(1:6));
P_mech_duct = sum(P_mech(7:8));
P_mech_ref = max(P_mech_main, 1e-6);
FM = Pideal / P_mech_ref;
EnergyRemain_Wh = max(0, battery_Wh * usable_ratio - Energy_Wh);
EnduranceRemain_h = EnergyRemain_Wh / max(P_elec_total, 1e-6);
speed_mps = sqrt(vel_world(1)^2 + vel_world(2)^2 + vel_world(3)^2);
RangeEstimate_km = speed_mps * 3.6 * EnduranceRemain_h;
perf_vec = zeros(20, 1);
perf_vec(1) = t;
perf_vec(2:9) = W(1:8);
perf_vec(10) = P_mech_main;
perf_vec(11) = P_mech_duct;
perf_vec(12) = P_elec_total;
perf_vec(13) = Energy_Wh;
perf_vec(14) = FM;
perf_vec(15) = DL;
perf_vec(16) = Sigma;
perf_vec(17) = Vi;
perf_vec(18) = speed_mps;
perf_vec(19) = EnduranceRemain_h;
perf_vec(20) = RangeEstimate_km;
end

== matlab function overalldesign_change_down/Optimization_Module/extract_metrics ==
  data: performance_output input; Energy_Wh output; P_elec_total_W output; EnduranceRemain_h output; RangeEstimate_km output; MaxRotorSpeed_radps output; OptimizationScore output; RouteModeCmd output; SpeedScale output; ThrustScale output; ControlScale output
function [Energy_Wh, P_elec_total_W, EnduranceRemain_h, RangeEstimate_km, MaxRotorSpeed_radps, OptimizationScore, RouteModeCmd, SpeedScale, ThrustScale, ControlScale] = extract_metrics(performance_output)
%#codegen
W = performance_output(2:9);
P_elec_total_W = performance_output(12);
Energy_Wh = performance_output(13);
EnduranceRemain_h = performance_output(19);
RangeEstimate_km = performance_output(20);
MaxRotorSpeed_radps = max(W);

speed_max_radps = 1770;
speed_high = 0.88 * speed_max_radps;
speed_critical = 0.97 * speed_max_radps;
rotor_stress = saturate((MaxRotorSpeed_radps - speed_high) / max(speed_critical - speed_high, 1e-6));
power_stress = saturate((P_elec_total_W - 220000) / max(350000 - 220000, 1e-6));
stress = max(rotor_stress, power_stress);

% Conservative online commands. The Memory blocks outside this module
% provide the one-step delay needed to avoid a direct algebraic loop.
t_route_s = performance_output(1);
if t_route_s < 64
    RouteModeCmd = 1;
elseif t_route_s < 1140
    RouteModeCmd = 3;
else
    RouteModeCmd = 5;
end
SpeedScale = 1 - 0.20 * stress;
ThrustScale = 1 - 0.05 * rotor_stress;
ControlScale = 1 - 0.25 * stress;

SpeedScale = min(1.05, max(0.75, SpeedScale));
ThrustScale = min(1.02, max(0.92, ThrustScale));
ControlScale = min(1.05, max(0.70, ControlScale));
OptimizationScore = Energy_Wh * (1 + 20 * rotor_stress^2);
end

function y = saturate(u)
y = min(1, max(0, u));
end

== matlab function overalldesign_change_down/Flight_Simulation/Dynamics_Subsys/Aero_Model/MATLAB Function ==
  data: V_body input; F_aero output; euler input; M_aero output
function [F_aero, M_aero] = aero_model(V_body, euler)
% 20 m/s forward-flight aero loads in model body axes, moment about CG.
% euler = [phi; theta; psi], rad

V_ref = 20.0;
V = sqrt(V_body(1)^2 + V_body(2)^2 + V_body(3)^2);

% Hover or very-low-speed: do not use 20 m/s aero data.
if V < 5
    F_aero = [0; 0; 0];
    M_aero = [0; 0; 0];
    return;
end

theta_deg = euler(2) * 180 / pi;
theta_deg = min(max(theta_deg, 0), 5);
lambda = theta_deg / 5;

F0 = [-872.34;   15.33;  -1788.918];
M0 = [  23.102; 2694.1325; 15.7031];

F5 = [-933.79;   -25.627; -1539.22];
M5 = [  68.8477; 2599.56;  61.048];

% Optional dynamic-pressure correction if speed drifts from 20 m/s.
q_scale = (V / V_ref)^2;

F_aero = q_scale * (F0 + lambda * (F5 - F0));
M_aero = q_scale * (M0 + lambda * (M5 - M0));
end

== matlab function overalldesign_change_down/Flight_Simulation/Dynamics_Subsys/motor_model ==
  data: W input; F_body output; M_body output; CGoffset input; motor_coord input
function [F_body, M_body] = motor_model(W, CGoffset, motor_coord)
% W(1:6) = rotor speed, W(7:8) = duct speed
% Change these two constants before each tilt case.
tilt_mode = 0;
tilt_deg = 0;

% tilt_mode:
%   0 = no tilt
%   1 = staggered X tilt: motors 1/4/5 +X, motors 2/3/6 -X
%   2 = inward Y tilt: motors 1/3/5 +Y, motors 2/4/6 -Y
%   3 = outward Y tilt: motors 1/3/5 -Y, motors 2/4/6 +Y

kF = 0.0013767;
kM = 0.000164967;
kF_duct = 4.54e-05;

motor_pos_0 = motor_coord(1:6, 1:3);
duct_pos_0 = motor_coord(7:8, 1:3);

motor_dir = [1; -1; -1; 1; 1; -1];
duct_dir = [0, -1, 0; 0, 1, 0];

motor_pos = motor_pos_0 - CGoffset';
duct_pos  = duct_pos_0  - CGoffset';

alpha = tilt_deg * pi / 180;

F_rotor_total = zeros(3, 1);
M_rotor_total = zeros(3, 1);

for i = 1:6
    Ti = kF * W(i)^2;

    if tilt_mode == 0
        hxy = [0, 0];

    elseif tilt_mode == 1
        if i == 1 || i == 4 || i == 5
            hxy = [1, 0];
        else
            hxy = [-1, 0];
        end

    elseif tilt_mode == 2
        if i == 1 || i == 3 || i == 5
            hxy = [0, 1];
        else
            hxy = [0, -1];
        end

    elseif tilt_mode == 3
        if i == 1 || i == 3 || i == 5
            hxy = [0, -1];
        else
            hxy = [0, 1];
        end

    else
        hxy = [0, 0];
    end

    thrust_dir = [sin(alpha) * hxy(1);
                  sin(alpha) * hxy(2);
                 -cos(alpha)];

    Fi = Ti * thrust_dir;
    ri = motor_pos(i, :)';

    Mi_force = cross(ri, Fi);
    Mi_react = motor_dir(i) * kM * W(i)^2 * (-thrust_dir);

    F_rotor_total = F_rotor_total + Fi;
    M_rotor_total = M_rotor_total + Mi_force + Mi_react;
end

F1 = kF_duct * W(7)^2;
F2 = kF_duct * W(8)^2;

F_duct_x = F1 * duct_dir(1, 1) + F2 * duct_dir(2, 1);
F_duct_y = F1 * duct_dir(1, 2) + F2 * duct_dir(2, 2);

F_duct_1 = [F1 * duct_dir(1, 1); F1 * duct_dir(1, 2); 0];
F_duct_2 = [F2 * duct_dir(2, 1); F2 * duct_dir(2, 2); 0];

tau_duct = cross(duct_pos(1, :)', F_duct_1) + ...
           cross(duct_pos(2, :)', F_duct_2);

F_body = F_rotor_total + [F_duct_x; F_duct_y; 0];
M_body = M_rotor_total + tau_duct;
end

== matlab function overalldesign_change_down/Flight_Simulation/rhs_to_unity ==
  data: pos_body input; data output; euler_body_rad input
function data = rhs_to_unity(pos_body, euler_body_rad)
pos_u = [pos_body(2); -pos_body(3); pos_body(1)];
euler_u_deg = [-euler_body_rad(2); euler_body_rad(3); -euler_body_rad(1)] * 180/pi;
data = [pos_u; euler_u_deg];
end

== matlab function overalldesign_change_down/Route_Manager/Accel_Descend/descend_profile ==
  data: t_clock input; z output; z0 input; V_descent input; a_brake input
function z = descend_profile(t_clock, z0, V_descent, a_brake)
t_peak = V_descent / a_brake;
if t_clock <= t_peak
    dz = 0.5 * a_brake * t_clock^2;
elseif t_clock <= 2 * t_peak
    dt = t_clock - t_peak;
    dz = 0.5 * a_brake * t_peak^2 + V_descent * dt - 0.5 * a_brake * dt^2;
else
    dz = V_descent * t_peak;
end
z = z0 + dz;
end

== matlab function overalldesign_change_down/Flight_Simulation/Dynamics_Subsys/GravBlock ==
  data: euler input; F_grav output
function F_grav = grav_block(euler)
% Gravity force in body frame (NED: Z down, gravity = +Z in world)
% g_body = DCM_be' * [0; 0; m*g]
g = 9.81; m = 1200;
phi = euler(1); theta = euler(2);
sp = sin(theta); cp = cos(theta);
sr = sin(phi); cr = cos(phi);
F_grav = m * g * [-sp; cp*sr; cp*cr];
end

== matlab function overalldesign_change_down/Flight_Simulation/controller/Accel2Attitude/accel2quat ==
  data: ax input; qw output; ay input; az input; psi input; qx output; qy output; qz output; thr output
function [qw, qx, qy, qz, thr] = accel2quat(ax, ay, az, psi)
g = 9.81; m = 1200;
norm_bz = sqrt((-ax)^2 + (-ay)^2 + (g-az)^2);
if norm_bz < 0.1; norm_bz = 0.1; end
T = m * norm_bz;
thr = max(0, min(20000, T));
bz_x = -ax / norm_bz;
bz_y = -ay / norm_bz;
bz_z = (g-az) / norm_bz;
max_tilt_rad = 20 * pi / 180;
horiz_norm = sqrt(bz_x^2 + bz_y^2);
max_horiz = sin(max_tilt_rad);
if horiz_norm > max_horiz
    scale = max_horiz / horiz_norm;
    bz_x = bz_x * scale; bz_y = bz_y * scale;
    bz_z = cos(max_tilt_rad);
end
hx = cos(psi); hy = sin(psi);
by_x = bz_y * 0 - bz_z * hy;
by_y = bz_z * hx - bz_x * 0;
by_z = bz_x * hy - bz_y * hx;
nby = sqrt(by_x^2 + by_y^2 + by_z^2);
if nby < 0.01
    by_x = 0; by_y = 1; by_z = 0;
else
    by_x = by_x / nby; by_y = by_y / nby; by_z = by_z / nby;
end
bx_x = by_y * bz_z - by_z * bz_y;
bx_y = by_z * bz_x - by_x * bz_z;
bx_z = by_x * bz_y - by_y * bz_x;
R11 = bx_x; R12 = by_x; R13 = bz_x;
R21 = bx_y; R22 = by_y; R23 = bz_y;
R31 = bx_z; R32 = by_z; R33 = bz_z;
tr = R11 + R22 + R33;
if tr > 0
    S = 2 * sqrt(tr + 1);
    qw = 0.25 * S;
    qx = (R32 - R23) / S;
    qy = (R13 - R31) / S;
    qz = (R21 - R12) / S;
elseif R11 > R22 && R11 > R33
    S = 2 * sqrt(1 + R11 - R22 - R33);
    qw = (R32 - R23) / S;
    qx = 0.25 * S;
    qy = (R12 + R21) / S;
    qz = (R13 + R31) / S;
elseif R22 > R33
    S = 2 * sqrt(1 + R22 - R11 - R33);
    qw = (R13 - R31) / S;
    qx = (R12 + R21) / S;
    qy = 0.25 * S;
    qz = (R23 + R32) / S;
else
    S = 2 * sqrt(1 + R33 - R11 - R22);
    qw = (R21 - R12) / S;
    qx = (R13 + R31) / S;
    qy = (R23 + R32) / S;
    qz = 0.25 * S;
end
qn = sqrt(qw^2 + qx^2 + qy^2 + qz^2);
qw = qw / qn; qx = qx / qn; qy = qy / qn; qz = qz / qn;
end

== matlab function overalldesign_change_down/Flight_Simulation/controller/Euler2Quat/euler2quat ==
  data: phi input; qw output; theta input; psi input; qx output; qy output; qz output
function [qw, qx, qy, qz] = euler2quat(phi, theta, psi)
cy = cos(psi/2); sy = sin(psi/2);
cp = cos(theta/2); sp = sin(theta/2);
cr = cos(phi/2); sr = sin(phi/2);
qw = cr*cp*cy + sr*sp*sy;
qx = sr*cp*cy - cr*sp*sy;
qy = cr*sp*cy + sr*cp*sy;
qz = cr*cp*sy - sr*sp*cy;
end

== matlab function overalldesign_change_down/Flight_Simulation/controller/Attitude_Controller/quat_att_control ==
  data: qw_des input; p_sp output; qx_des input; qy_des input; qz_des input; qw_cur input; qx_cur input; qy_cur input; qz_cur input; q_sp output; r_sp output
function [p_sp, q_sp, r_sp] = quat_att_control(qw_des, qx_des, qy_des, qz_des, qw_cur, qx_cur, qy_cur, qz_cur)
% PX4-style reduced attitude control in NED right-handed frame
% Step 1: body-Z axes in inertial frame
Kp_tilt = 1.5; Kp_yaw = 1.2; k_yaw_weight = 0.7;
bz_cur_x = 2*(qw_cur*qy_cur + qx_cur*qz_cur);
bz_cur_y = 2*(qy_cur*qz_cur - qw_cur*qx_cur);
bz_cur_z = qw_cur^2 - qx_cur^2 - qy_cur^2 + qz_cur^2;
bz_des_x = 2*(qw_des*qy_des + qx_des*qz_des);
bz_des_y = 2*(qy_des*qz_des - qw_des*qx_des);
bz_des_z = qw_des^2 - qx_des^2 - qy_des^2 + qz_des^2;
% Step 2: tilt error rotation axis k = bz_cur x bz_des (inertial frame)
k_x = bz_cur_y*bz_des_z - bz_cur_z*bz_des_y;
k_y = bz_cur_z*bz_des_x - bz_cur_x*bz_des_z;
k_z = bz_cur_x*bz_des_y - bz_cur_y*bz_des_x;
k_norm = sqrt(k_x^2 + k_y^2 + k_z^2);
cos_theta = bz_cur_x*bz_des_x + bz_cur_y*bz_des_y + bz_cur_z*bz_des_z;
cos_theta = max(-1.0, min(1.0, cos_theta));
theta = acos(cos_theta);
% Step 3: qer = tilt error quaternion (inertial frame)
if k_norm < 1e-6
    qer_w = 1.0; qer_x = 0.0; qer_y = 0.0; qer_z = 0.0;
else
    k_hat_x = k_x / k_norm; k_hat_y = k_y / k_norm; k_hat_z = k_z / k_norm;
    sin_half = sin(theta / 2);
    qer_w = cos(theta / 2);
    qer_x = k_hat_x * sin_half;
    qer_y = k_hat_y * sin_half;
    qer_z = k_hat_z * sin_half;
end
% Step 4: qr = qer * q_cur (tilt-corrected attitude, inertial frame)
qr_w = qer_w*qw_cur - qer_x*qx_cur - qer_y*qy_cur - qer_z*qz_cur;
qr_x = qer_w*qx_cur + qer_x*qw_cur + qer_y*qz_cur - qer_z*qy_cur;
qr_y = qer_w*qy_cur - qer_x*qz_cur + qer_y*qw_cur + qer_z*qx_cur;
qr_z = qer_w*qz_cur + qer_x*qy_cur - qer_y*qx_cur + qer_z*qw_cur;
% Step 5: qme = qr* * q_des (remaining error = yaw only)
qme_w = qr_w*qw_des + qr_x*qx_des + qr_y*qy_des + qr_z*qz_des;
qme_x = qr_w*qx_des - qr_x*qw_des - qr_y*qz_des + qr_z*qy_des;
qme_y = qr_w*qy_des + qr_x*qz_des - qr_y*qw_des - qr_z*qx_des;
qme_z = qr_w*qz_des - qr_x*qy_des + qr_y*qx_des - qr_z*qw_des;
% Step 6: yaw correction quaternion qy = [cos(alpha/2), 0, 0, sin(alpha/2)]
alpha = 2 * atan2(qme_z, qme_w);
half_alpha = k_yaw_weight * alpha / 2;
qy_w = cos(half_alpha); qy_z = sin(half_alpha);
% Step 7: qm = qr * qy (full desired attitude with tilt+yaw correction)
qm_w = qr_w*qy_w - qr_z*qy_z;
qm_x = qr_x*qy_w + qr_y*qy_z;
qm_y = qr_y*qy_w - qr_x*qy_z;
qm_z = qr_z*qy_w + qr_w*qy_z;
% Step 8: qe = q_cur* * qm (ERROR IN BODY FRAME — key transformation!)
qe_w = qw_cur*qm_w + qx_cur*qm_x + qy_cur*qm_y + qz_cur*qm_z;
qe_x = qw_cur*qm_x - qx_cur*qm_w - qy_cur*qm_z + qz_cur*qm_y;
qe_y = qw_cur*qm_y + qx_cur*qm_z - qy_cur*qm_w - qz_cur*qm_x;
qe_z = qw_cur*qm_z - qx_cur*qm_y + qy_cur*qm_x - qz_cur*qm_w;
% Ensure shortest rotation
if qe_w < 0
    qe_x = -qe_x; qe_y = -qe_y; qe_z = -qe_z;
end

% Safety clamp: limit attitude error to prevent rate controller divergence
% qe_xyz = sin(theta/2)*axis, so max_qe=0.35 limits attitude error to ~40°
max_qe = 0.30;
qe_x = max(-max_qe, min(max_qe, qe_x));
qe_y = max(-max_qe, min(max_qe, qe_y));
qe_z = max(-max_qe, min(max_qe, qe_z));% Step 9: body-frame angular rate commands
% For small angles, qe_xyz = sin(theta/2)*axis ≈ theta/2 * axis
% So p_sp = Kp * 2 * qe_x = Kp * axis_x * theta
p_sp = max(-3.0, min(3.0, Kp_tilt * 2 * qe_x));
q_sp = max(-3.0, min(3.0, Kp_tilt * 2 * qe_y));
r_sp = max(-2.0, min(2.0, Kp_yaw * 2 * qe_z));
end
